simulink model "es3"  (R2022b)
settings: Solver=VariableStepAuto  StartTime=0.0  StopTime=10.0  RelTol=1e-3
undefined symbols (not defined in the file): A0, B0, C0, D0, den, DiscIntNeverNeededParam, K, Ki, Nu, num, Nx, sysD, Ts
settings Model: Creator=emanuelevitetta  LastModifiedBy=emanuelevitetta

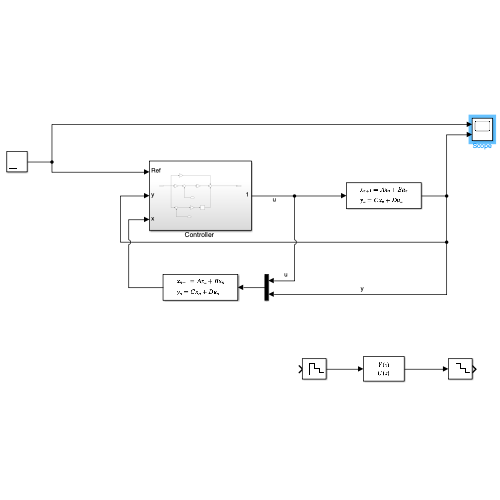
[thumbnail: Simulink's stored preview of the top-level diagram]
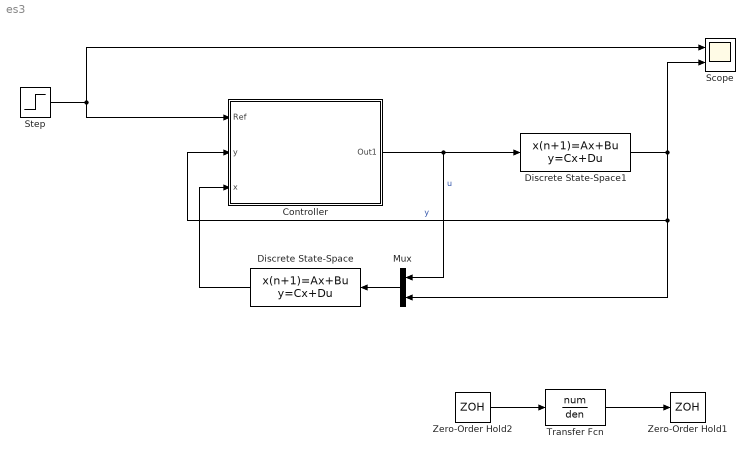
== system es3 ==
  "Controller " : Subsystem
  Discrete State-Space : DiscreteStateSpace  A=A0  B=B0  C=C0  D=D0  SampleTime=Ts
  Discrete State-Space1 : DiscreteStateSpace  A=sysD.A  B=sysD.B  C=sysD.C  D=sysD.D  SampleTime=-1
  Mux : Mux  Inputs=2
  Scope : Scope  NumInputPorts=2
  Step : Step  SampleTime=0
  Transfer Fcn : TransferFcn  Numerator=num  Denominator=den
  Zero-Order Hold1 : ZeroOrderHold  SampleTime=Ts
  Zero-Order Hold2 : ZeroOrderHold  SampleTime=Ts
  wires:
  Step/1 -> "Controller "/1(Ref), Scope/1
  Discrete State-Space/1 -> "Controller "/3(x)
  "Controller "/1(Out1) -> Mux/1, Discrete State-Space1/1  "u"
  Mux/1 -> Discrete State-Space/1
  Discrete State-Space1/1 -> "Controller "/2(y), Mux/2, Scope/2  "y"
  Transfer Fcn/1 -> Zero-Order Hold1/1
  Zero-Order Hold2/1 -> Transfer Fcn/1

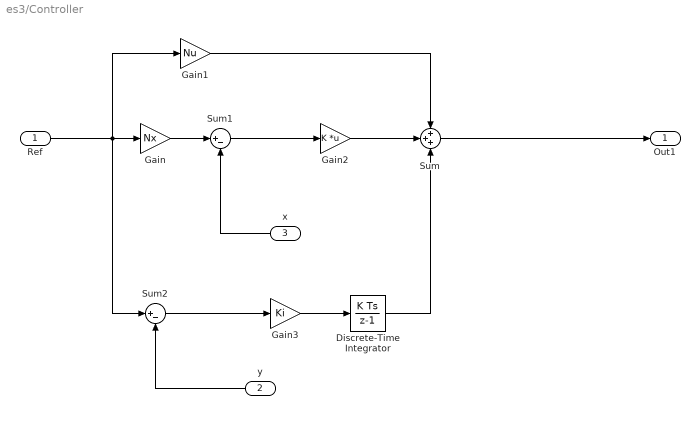
== system es3/Controller  ==
  Ref : Inport
  y : Inport  Port=2
  x : Inport  Port=3
  Discrete-Time Integrator : DiscreteIntegrator  SampleTime=Ts  ICPrevOutput=DiscIntNeverNeededParam  ICPrevScaledInput=DiscIntNeverNeededParam
  Gain : Gain  Gain=Nx
  Gain1 : Gain  Gain=Nu
  Gain2 : Gain  Gain=K  Multiplication=Matrix(K*u)
  Gain3 : Gain  Gain=Ki
  Sum : Sum  Inputs=+++
  Sum1 : Sum  Inputs=|+-
  Sum2 : Sum  Inputs=|+-
  Out1 : Outport
  wires:
  Ref/1 -> Sum2/1, Gain1/1, Gain/1
  Gain2/1 -> Sum/2
  Gain1/1 -> Sum/1
  Gain3/1 -> Discrete-Time Integrator/1
  Discrete-Time Integrator/1 -> Sum/3
  Sum1/1 -> Gain2/1
  Gain/1 -> Sum1/1
  Sum2/1 -> Gain3/1
  x/1 -> Sum1/2
  y/1 -> Sum2/2
  Sum/1 -> Out1/1
